simulink model "Uebung5_A3"  (R2016a)
settings: Solver=VariableStepAuto  StartTime=0.0  StopTime=100000  RelTol=1e-3
undefined symbols (not defined in the file or in its folder): m, n
settings Model: Creator=gome  LastModifiedBy=gome

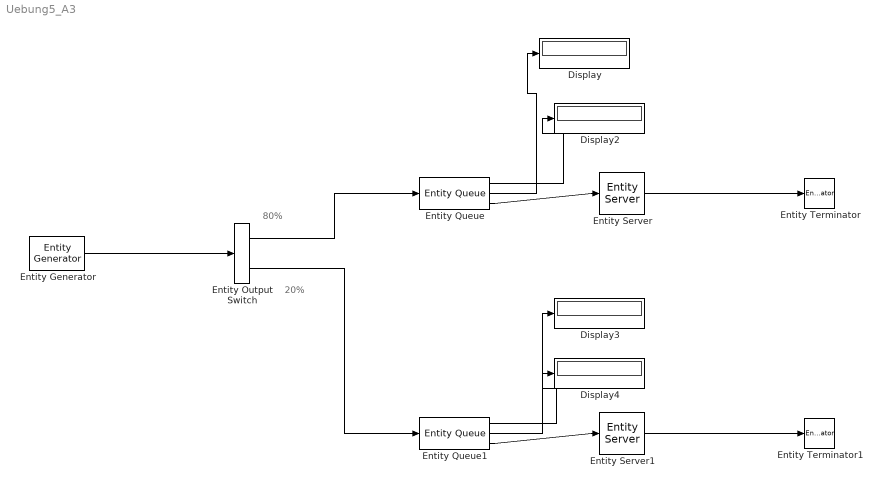
== system Uebung5_A3 ==
  note: 20%
  note: 80%
  Display{,2..4} (4 alike) : Display
  Entity Output Switch : EntityOutputSwitch  InputPortMessageModes=m  OutputPortMessageModes=m,m  SwitchingCriterion=From attribute  SwitchAttributeName=portNumber
  Entity Generator : EntityGenerator  OutputPortMessageModes=m  GenerateAction=entity.portNumber = binornd(1, 0.2) + 1;  AttributeName=portNumber  EntityType=Structured  EntityTypeName=Entity
  Entity Queue : EntityQueue  InputPortMessageModes=m  OutputPortMessageModes=n,n,m  Capacity=inf  AverageWait=on  AverageQueueLength=on
      settings: OutputPortMap=o2,o3,o5
  Entity Queue1 : EntityQueue  InputPortMessageModes=m  OutputPortMessageModes=n,n,m  Capacity=inf  AverageWait=on  AverageQueueLength=on
      settings: OutputPortMap=o2,o3,o5
  Entity Server : EntityServer  InputPortMessageModes=m  OutputPortMessageModes=m  Capacity=1  ServiceTimeValue=1.2
  Entity Server1 : EntityServer  InputPortMessageModes=m  OutputPortMessageModes=m  Capacity=1  ServiceTimeValue=4
  Entity Terminator : EntityTerminator  InputPortMessageModes=m
  Entity Terminator1 : EntityTerminator  InputPortMessageModes=m
  wires:
  Entity Generator/1 -> Entity Output Switch/1
  Entity Output Switch/1 -> Entity Queue/1
  Entity Output Switch/2 -> Entity Queue1/1
  Entity Queue/3 -> Entity Server/1
  Entity Queue1/3 -> Entity Server1/1
  Entity Server/1 -> Entity Terminator/1
  Entity Server1/1 -> Entity Terminator1/1
  Entity Queue/2 -> Display/1
  Entity Queue1/2 -> Display3/1
  Entity Queue1/1 -> Display4/1
  Entity Queue/1 -> Display2/1
